simulink model "DR18E_Testpult"  (R2017a)
settings: Solver=ode1  StartTime=0.0  StopTime=Inf  FixedStep=0.001  RelTol=1e-3
PostLoadFcn:
  | , if any(exist('dsrtsu_mdlpostloadfcn', 'file') == [2, 3, 6]), try dsrtsu_mdlpostloadfcn('Execute', bdroot); catch fprintf('Error in PostLoadFcn (dsrtsu_mdlpostloadfcn) for model "%s":\n %s\n', bdroot, lasterr); end, end,
model workspace: external: MAT-File C:\Users\DeltaRacing\Documents\dSPACE\MABX_DR18E\Model\DR18E_MABX_Parameter.mat (data not in the file)
values from neighbouring files (symbols this model uses):
  am = 1/Ts    (= 1)    [DR18E_MABX_Parameter.m]
  bm = K/Ts    (= 0.05)    [DR18E_MABX_Parameter.m]
  cf = 41350    [DR18E_MABX_Parameter.m]
  cr = 41350    [DR18E_MABX_Parameter.m]
  Derating_HV_Battery_Kapa = 1    [DR18E_MABX_Parameter.m]
  Derating_Start_km = 16    [DR18E_MABX_Parameter.m]
  Drive_Mode = 0    [DR18E_MABX_Parameter.m]
  g = 1    [DR18E_MABX_Parameter.m]
  Gas_Modus = 2    [DR18E_MABX_Parameter.m]
  HV_Power_max = 80    [DR18E_MABX_Parameter.m]
  i_Getriebe = 3.3    [DR18E_MABX_Parameter.m]
  i_Lenkgetriebe = 4.32    [DR18E_MABX_Parameter.m]
  K_SET = 1    [DR18E_MABX_Parameter.m]
  Kapazitaet_HV_Battery_kWh = 6.6    [DR18E_MABX_Parameter.m]
  KW_T_Soll = 37    [DR18E_MABX_Parameter.m]
  lf = 1.2    [DR18E_MABX_Parameter.m]
  lr = 1.15    [DR18E_MABX_Parameter.m]
  m = mdriver + mvehicle    (= 310)    [DR18E_MABX_Parameter.m]
  M_max = 150    [DR18E_MABX_Parameter.m]
  Power_Limit_onoff = 0    [DR18E_MABX_Parameter.m]
  Reifenradius = 0.2351    [DR18E_MABX_Parameter.m]
  Strecke_Endu_km = 22    [DR18E_MABX_Parameter.m]
  TC_Decr_Gas = 0.00005    (= 5e-05)    [DR18E_MABX_Parameter.m]
  TC_Derivative = 0.4    [DR18E_MABX_Parameter.m]
  TC_Incr_Gas = 0.005    [DR18E_MABX_Parameter.m]
  TC_On = 0    [DR18E_MABX_Parameter.m]
  TC_Relay_Off = 0.065    [DR18E_MABX_Parameter.m]
  TC_Relay_On = 0.07    [DR18E_MABX_Parameter.m]
  TV_Mode = 2    [DR18E_MABX_Parameter.m]
  TV_On = 0    [DR18E_MABX_Parameter.m]
  TV_Override = 1    [DR18E_MABX_Parameter.m]
  y = 0.8    [DR18E_MABX_Parameter.m]
undefined symbols (not defined in the file or in its folder): D, DiscIntNeverNeededParam, I, K_OL, P
libraries: simulink x288, rtican x100, rtiusbflightreclib x40, rti1401lib_dio_type3 x10, simulink_extras x10, rti1401lib_adc_type4 x8, rti1401lib_II_base x7
(part 17 of 27)

== system DR18E_Testpult/Verarbeitung/Precalculations/FlightRecorder ==
  In1 : Inport
  Data Type Conversion : DataTypeConversion
  Gain : Gain
  USB_FLIGHT_REC_BL1 : rtiusbflightreclib/USB_FLIGHT_REC_BL1  VarName=v_kmh  DataType=Single  SampleTime=-1  TLCFileName=rtiusbflightrecwrite  Reserved1=[]  Reserved2=[]  Reserved3=[]  Reserved4=[]  DSProperties=struct('RTI',struct('Version',uint32(3),'BlockType',struct('isSLSource',uint8(0),'isSLSink',uint8(1),'isHWSource',uint8(0),'isHWSink',uint8(0),'isSetup',uint8(0),'isInline',uint8(1),'isNonInline',uint8(0),'isInterrupt',uint8(0),'isChannelwise',uint8(0)),'IOBoardType',{{'DSUSB','FLIGHTREC'}},'UnitType','FLIGHTREC','Identifier','WRITE','DialogType','SL','BlockSet','RTIUSBFLIGHTREC','SlaveProcessor','NONE'))  RTIBlockInterface=struct('InputPortsActive',1,'InputPortsWidth',int32(1),'InputPortsDataType',{{'SS_SINGLE'}},'BlockDisplay',{{['Write to\nUSB Flight Recorder'],'center'}},'IconTransparency','off','InitLevel',3,'BlockName',struct('Token',{{'USB_FLIGHT_REC_BL1'}}),'MaskDescription',['Write input to the Flight Recorder. Recorded data can be referenced by the specified variable.'],'SampleTime',{{-1}})  RTIBlockParameters=struct('VarName',{{'v_kmh','OFF',[]}},'DataType',{{'Single','OFF',[]}},'SampleTime',{{-1,'OFF',[]}},'TLCFileName',{{'rtiusbflightrecwrite','OFF',[]}})  RTISFcnParameters=struct('VarName','char','DataType','char','SampleTime','double','TLCFileName','char')  RTIBlockParaDefault=struct('VarName','Var1','DataType','Single','SampleTime',-1,'TLCFileName','rtiusbflightrecwrite')
      settings: SourceProductName=dSPACE RTI USB Flight Rec Blockset
  wires:
  Data Type Conversion/1 -> USB_FLIGHT_REC_BL1/1
  In1/1 -> Gain/1
  Gain/1 -> Data Type Conversion/1

== system DR18E_Testpult/Verarbeitung/Precalculations/FlightRecorder1 ==
  In1 : Inport
  Data Type Conversion : DataTypeConversion
  Gain : Gain
  USB_FLIGHT_REC_BL1 : rtiusbflightreclib/USB_FLIGHT_REC_BL1  VarName=DrehzahlRL_rpm  DataType=Single  SampleTime=-1  TLCFileName=rtiusbflightrecwrite  Reserved1=[]  Reserved2=[]  Reserved3=[]  Reserved4=[]  DSProperties=struct('RTI',struct('Version',uint32(3),'BlockType',struct('isSLSource',uint8(0),'isSLSink',uint8(1),'isHWSource',uint8(0),'isHWSink',uint8(0),'isSetup',uint8(0),'isInline',uint8(1),'isNonInline',uint8(0),'isInterrupt',uint8(0),'isChannelwise',uint8(0)),'IOBoardType',{{'DSUSB','FLIGHTREC'}},'UnitType','FLIGHTREC','Identifier','WRITE','DialogType','SL','BlockSet','RTIUSBFLIGHTREC','SlaveProcessor','NONE'))  RTIBlockInterface=struct('InputPortsActive',1,'InputPortsWidth',int32(1),'InputPortsDataType',{{'SS_SINGLE'}},'BlockDisplay',{{['Write to\nUSB Flight Recorder'],'center'}},'IconTransparency','off','InitLevel',3,'BlockName',struct('Token',{{'USB_FLIGHT_REC_BL1'}}),'MaskDescription',['Write input to the Flight Recorder. Recorded data can be referenced by the specified variable.'],'SampleTime',{{-1}})  RTIBlockParameters=struct('VarName',{{'DrehzahlRL_rpm','OFF',[]}},'DataType',{{'Single','OFF',[]}},'SampleTime',{{-1,'OFF',[]}},'TLCFileName',{{'rtiusbflightrecwrite','OFF',[]}})  RTISFcnParameters=struct('VarName','char','DataType','char','SampleTime','double','TLCFileName','char')  RTIBlockParaDefault=struct('VarName','Var1','DataType','Single','SampleTime',-1,'TLCFileName','rtiusbflightrecwrite')
      settings: SourceProductName=dSPACE RTI USB Flight Rec Blockset
  wires:
  Data Type Conversion/1 -> USB_FLIGHT_REC_BL1/1
  In1/1 -> Gain/1
  Gain/1 -> Data Type Conversion/1

== system DR18E_Testpult/Verarbeitung/Precalculations/FlightRecorder2 ==
  In1 : Inport
  Data Type Conversion : DataTypeConversion
  Gain : Gain
  USB_FLIGHT_REC_BL1 : rtiusbflightreclib/USB_FLIGHT_REC_BL1  VarName=DrehzahlRR_rpm  DataType=Single  SampleTime=-1  TLCFileName=rtiusbflightrecwrite  Reserved1=[]  Reserved2=[]  Reserved3=[]  Reserved4=[]  DSProperties=struct('RTI',struct('Version',uint32(3),'BlockType',struct('isSLSource',uint8(0),'isSLSink',uint8(1),'isHWSource',uint8(0),'isHWSink',uint8(0),'isSetup',uint8(0),'isInline',uint8(1),'isNonInline',uint8(0),'isInterrupt',uint8(0),'isChannelwise',uint8(0)),'IOBoardType',{{'DSUSB','FLIGHTREC'}},'UnitType','FLIGHTREC','Identifier','WRITE','DialogType','SL','BlockSet','RTIUSBFLIGHTREC','SlaveProcessor','NONE'))  RTIBlockInterface=struct('InputPortsActive',1,'InputPortsWidth',int32(1),'InputPortsDataType',{{'SS_SINGLE'}},'BlockDisplay',{{['Write to\nUSB Flight Recorder'],'center'}},'IconTransparency','off','InitLevel',3,'BlockName',struct('Token',{{'USB_FLIGHT_REC_BL1'}}),'MaskDescription',['Write input to the Flight Recorder. Recorded data can be referenced by the specified variable.'],'SampleTime',{{-1}})  RTIBlockParameters=struct('VarName',{{'DrehzahlRR_rpm','OFF',[]}},'DataType',{{'Single','OFF',[]}},'SampleTime',{{-1,'OFF',[]}},'TLCFileName',{{'rtiusbflightrecwrite','OFF',[]}})  RTISFcnParameters=struct('VarName','char','DataType','char','SampleTime','double','TLCFileName','char')  RTIBlockParaDefault=struct('VarName','Var1','DataType','Single','SampleTime',-1,'TLCFileName','rtiusbflightrecwrite')
      settings: SourceProductName=dSPACE RTI USB Flight Rec Blockset
  wires:
  Data Type Conversion/1 -> USB_FLIGHT_REC_BL1/1
  In1/1 -> Gain/1
  Gain/1 -> Data Type Conversion/1

== system DR18E_Testpult/Verarbeitung/Precalculations/FlightRecorder3 ==
  In1 : Inport
  Data Type Conversion : DataTypeConversion
  Gain : Gain
  USB_FLIGHT_REC_BL1 : rtiusbflightreclib/USB_FLIGHT_REC_BL1  VarName=DrehzahlFR_rpm  DataType=Single  SampleTime=-1  TLCFileName=rtiusbflightrecwrite  Reserved1=[]  Reserved2=[]  Reserved3=[]  Reserved4=[]  DSProperties=struct('RTI',struct('Version',uint32(3),'BlockType',struct('isSLSource',uint8(0),'isSLSink',uint8(1),'isHWSource',uint8(0),'isHWSink',uint8(0),'isSetup',uint8(0),'isInline',uint8(1),'isNonInline',uint8(0),'isInterrupt',uint8(0),'isChannelwise',uint8(0)),'IOBoardType',{{'DSUSB','FLIGHTREC'}},'UnitType','FLIGHTREC','Identifier','WRITE','DialogType','SL','BlockSet','RTIUSBFLIGHTREC','SlaveProcessor','NONE'))  RTIBlockInterface=struct('InputPortsActive',1,'InputPortsWidth',int32(1),'InputPortsDataType',{{'SS_SINGLE'}},'BlockDisplay',{{['Write to\nUSB Flight Recorder'],'center'}},'IconTransparency','off','InitLevel',3,'BlockName',struct('Token',{{'USB_FLIGHT_REC_BL1'}}),'MaskDescription',['Write input to the Flight Recorder. Recorded data can be referenced by the specified variable.'],'SampleTime',{{-1}})  RTIBlockParameters=struct('VarName',{{'DrehzahlFR_rpm','OFF',[]}},'DataType',{{'Single','OFF',[]}},'SampleTime',{{-1,'OFF',[]}},'TLCFileName',{{'rtiusbflightrecwrite','OFF',[]}})  RTISFcnParameters=struct('VarName','char','DataType','char','SampleTime','double','TLCFileName','char')  RTIBlockParaDefault=struct('VarName','Var1','DataType','Single','SampleTime',-1,'TLCFileName','rtiusbflightrecwrite')
      settings: SourceProductName=dSPACE RTI USB Flight Rec Blockset
  wires:
  Data Type Conversion/1 -> USB_FLIGHT_REC_BL1/1
  In1/1 -> Gain/1
  Gain/1 -> Data Type Conversion/1

== system DR18E_Testpult/Verarbeitung/Precalculations/FlightRecorder4 ==
  In1 : Inport
  Data Type Conversion : DataTypeConversion
  Gain : Gain
  USB_FLIGHT_REC_BL1 : rtiusbflightreclib/USB_FLIGHT_REC_BL1  VarName=DrehzahlFL_rpm  DataType=Single  SampleTime=-1  TLCFileName=rtiusbflightrecwrite  Reserved1=[]  Reserved2=[]  Reserved3=[]  Reserved4=[]  DSProperties=struct('RTI',struct('Version',uint32(3),'BlockType',struct('isSLSource',uint8(0),'isSLSink',uint8(1),'isHWSource',uint8(0),'isHWSink',uint8(0),'isSetup',uint8(0),'isInline',uint8(1),'isNonInline',uint8(0),'isInterrupt',uint8(0),'isChannelwise',uint8(0)),'IOBoardType',{{'DSUSB','FLIGHTREC'}},'UnitType','FLIGHTREC','Identifier','WRITE','DialogType','SL','BlockSet','RTIUSBFLIGHTREC','SlaveProcessor','NONE'))  RTIBlockInterface=struct('InputPortsActive',1,'InputPortsWidth',int32(1),'InputPortsDataType',{{'SS_SINGLE'}},'BlockDisplay',{{['Write to\nUSB Flight Recorder'],'center'}},'IconTransparency','off','InitLevel',3,'BlockName',struct('Token',{{'USB_FLIGHT_REC_BL1'}}),'MaskDescription',['Write input to the Flight Recorder. Recorded data can be referenced by the specified variable.'],'SampleTime',{{-1}})  RTIBlockParameters=struct('VarName',{{'DrehzahlFL_rpm','OFF',[]}},'DataType',{{'Single','OFF',[]}},'SampleTime',{{-1,'OFF',[]}},'TLCFileName',{{'rtiusbflightrecwrite','OFF',[]}})  RTISFcnParameters=struct('VarName','char','DataType','char','SampleTime','double','TLCFileName','char')  RTIBlockParaDefault=struct('VarName','Var1','DataType','Single','SampleTime',-1,'TLCFileName','rtiusbflightrecwrite')
      settings: SourceProductName=dSPACE RTI USB Flight Rec Blockset
  wires:
  Data Type Conversion/1 -> USB_FLIGHT_REC_BL1/1
  In1/1 -> Gain/1
  Gain/1 -> Data Type Conversion/1

== system DR18E_Testpult/Verarbeitung/Precalculations/FlightRecorder5 ==
  In1 : Inport
  Data Type Conversion : DataTypeConversion
  Gain : Gain
  USB_FLIGHT_REC_BL1 : rtiusbflightreclib/USB_FLIGHT_REC_BL1  VarName=slip_links_0_1  DataType=Single  SampleTime=-1  TLCFileName=rtiusbflightrecwrite  Reserved1=[]  Reserved2=[]  Reserved3=[]  Reserved4=[]  DSProperties=struct('RTI',struct('Version',uint32(3),'BlockType',struct('isSLSource',uint8(0),'isSLSink',uint8(1),'isHWSource',uint8(0),'isHWSink',uint8(0),'isSetup',uint8(0),'isInline',uint8(1),'isNonInline',uint8(0),'isInterrupt',uint8(0),'isChannelwise',uint8(0)),'IOBoardType',{{'DSUSB','FLIGHTREC'}},'UnitType','FLIGHTREC','Identifier','WRITE','DialogType','SL','BlockSet','RTIUSBFLIGHTREC','SlaveProcessor','NONE'))  RTIBlockInterface=struct('InputPortsActive',1,'InputPortsWidth',int32(1),'InputPortsDataType',{{'SS_SINGLE'}},'BlockDisplay',{{['Write to\nUSB Flight Recorder'],'center'}},'IconTransparency','off','InitLevel',3,'BlockName',struct('Token',{{'USB_FLIGHT_REC_BL1'}}),'MaskDescription',['Write input to the Flight Recorder. Recorded data can be referenced by the specified variable.'],'SampleTime',{{-1}})  RTIBlockParameters=struct('VarName',{{'slip_links_0_1','OFF',[]}},'DataType',{{'Single','OFF',[]}},'SampleTime',{{-1,'OFF',[]}},'TLCFileName',{{'rtiusbflightrecwrite','OFF',[]}})  RTISFcnParameters=struct('VarName','char','DataType','char','SampleTime','double','TLCFileName','char')  RTIBlockParaDefault=struct('VarName','Var1','DataType','Single','SampleTime',-1,'TLCFileName','rtiusbflightrecwrite')
      settings: SourceProductName=dSPACE RTI USB Flight Rec Blockset
  wires:
  Data Type Conversion/1 -> USB_FLIGHT_REC_BL1/1
  In1/1 -> Gain/1
  Gain/1 -> Data Type Conversion/1

== system DR18E_Testpult/Verarbeitung/Precalculations/FlightRecorder6 ==
  In1 : Inport
  Data Type Conversion : DataTypeConversion
  Gain : Gain
  USB_FLIGHT_REC_BL1 : rtiusbflightreclib/USB_FLIGHT_REC_BL1  VarName=slip_rechts_0_1  DataType=Single  SampleTime=-1  TLCFileName=rtiusbflightrecwrite  Reserved1=[]  Reserved2=[]  Reserved3=[]  Reserved4=[]  DSProperties=struct('RTI',struct('Version',uint32(3),'BlockType',struct('isSLSource',uint8(0),'isSLSink',uint8(1),'isHWSource',uint8(0),'isHWSink',uint8(0),'isSetup',uint8(0),'isInline',uint8(1),'isNonInline',uint8(0),'isInterrupt',uint8(0),'isChannelwise',uint8(0)),'IOBoardType',{{'DSUSB','FLIGHTREC'}},'UnitType','FLIGHTREC','Identifier','WRITE','DialogType','SL','BlockSet','RTIUSBFLIGHTREC','SlaveProcessor','NONE'))  RTIBlockInterface=struct('InputPortsActive',1,'InputPortsWidth',int32(1),'InputPortsDataType',{{'SS_SINGLE'}},'BlockDisplay',{{['Write to\nUSB Flight Recorder'],'center'}},'IconTransparency','off','InitLevel',3,'BlockName',struct('Token',{{'USB_FLIGHT_REC_BL1'}}),'MaskDescription',['Write input to the Flight Recorder. Recorded data can be referenced by the specified variable.'],'SampleTime',{{-1}})  RTIBlockParameters=struct('VarName',{{'slip_rechts_0_1','OFF',[]}},'DataType',{{'Single','OFF',[]}},'SampleTime',{{-1,'OFF',[]}},'TLCFileName',{{'rtiusbflightrecwrite','OFF',[]}})  RTISFcnParameters=struct('VarName','char','DataType','char','SampleTime','double','TLCFileName','char')  RTIBlockParaDefault=struct('VarName','Var1','DataType','Single','SampleTime',-1,'TLCFileName','rtiusbflightrecwrite')
      settings: SourceProductName=dSPACE RTI USB Flight Rec Blockset
  wires:
  Data Type Conversion/1 -> USB_FLIGHT_REC_BL1/1
  In1/1 -> Gain/1
  Gain/1 -> Data Type Conversion/1

== system DR18E_Testpult/Verarbeitung/Precalculations/kilometer tracking ==
  v_ms : Inport
  Discrete-Time Integrator : DiscreteIntegrator  SampleTime=-1  ICPrevOutput=DiscIntNeverNeededParam  ICPrevScaledInput=DiscIntNeverNeededParam
  FlightRecorder1 : Subsystem
  s_m : Gain
  tag scope: Tagesmeter_s_m=global
  wires:
  v_ms/1 -> Discrete-Time Integrator/1
  s_m/1 -> [Tagesmeter_s_m], FlightRecorder1/1(In1)  "Tagesmeter_fluechtig_s_m"
  Discrete-Time Integrator/1 -> s_m/1

== system DR18E_Testpult/Verarbeitung/Strom//SOC/HVIRecorder ==
  In1 : Inport
  Data Type Conversion : DataTypeConversion
  Gain : Gain
  USB_FLIGHT_REC_BL1 : rtiusbflightreclib/USB_FLIGHT_REC_BL1  VarName=HV_current_A  DataType=Single  SampleTime=-1  TLCFileName=rtiusbflightrecwrite  Reserved1=[]  Reserved2=[]  Reserved3=[]  Reserved4=[]  DSProperties=struct('RTI',struct('Version',uint32(3),'BlockType',struct('isSLSource',uint8(0),'isSLSink',uint8(1),'isHWSource',uint8(0),'isHWSink',uint8(0),'isSetup',uint8(0),'isInline',uint8(1),'isNonInline',uint8(0),'isInterrupt',uint8(0),'isChannelwise',uint8(0)),'IOBoardType',{{'DSUSB','FLIGHTREC'}},'UnitType','FLIGHTREC','Identifier','WRITE','DialogType','SL','BlockSet','RTIUSBFLIGHTREC','SlaveProcessor','NONE'))  RTIBlockInterface=struct('InputPortsActive',1,'InputPortsWidth',int32(1),'InputPortsDataType',{{'SS_SINGLE'}},'BlockDisplay',{{['Write to\nUSB Flight Recorder'],'center'}},'IconTransparency','off','InitLevel',3,'BlockName',struct('Token',{{'USB_FLIGHT_REC_BL1'}}),'MaskDescription',['Write input to the Flight Recorder. Recorded data can be referenced by the specified variable.'],'SampleTime',{{-1}})  RTIBlockParameters=struct('VarName',{{'HV_current_A','OFF',[]}},'DataType',{{'Single','OFF',[]}},'SampleTime',{{-1,'OFF',[]}},'TLCFileName',{{'rtiusbflightrecwrite','OFF',[]}})  RTISFcnParameters=struct('VarName','char','DataType','char','SampleTime','double','TLCFileName','char')  RTIBlockParaDefault=struct('VarName','Var1','DataType','Single','SampleTime',-1,'TLCFileName','rtiusbflightrecwrite')
      settings: SourceProductName=dSPACE RTI USB Flight Rec Blockset
  wires:
  Data Type Conversion/1 -> USB_FLIGHT_REC_BL1/1
  In1/1 -> Gain/1
  Gain/1 -> Data Type Conversion/1

== system DR18E_Testpult/Verarbeitung/Strom//SOC/HVURecorder ==
  In1 : Inport
  Data Type Conversion : DataTypeConversion
  Gain : Gain
  USB_FLIGHT_REC_BL1 : rtiusbflightreclib/USB_FLIGHT_REC_BL1  VarName=HV_voltage_V  DataType=Single  SampleTime=-1  TLCFileName=rtiusbflightrecwrite  Reserved1=[]  Reserved2=[]  Reserved3=[]  Reserved4=[]  DSProperties=struct('RTI',struct('Version',uint32(3),'BlockType',struct('isSLSource',uint8(0),'isSLSink',uint8(1),'isHWSource',uint8(0),'isHWSink',uint8(0),'isSetup',uint8(0),'isInline',uint8(1),'isNonInline',uint8(0),'isInterrupt',uint8(0),'isChannelwise',uint8(0)),'IOBoardType',{{'DSUSB','FLIGHTREC'}},'UnitType','FLIGHTREC','Identifier','WRITE','DialogType','SL','BlockSet','RTIUSBFLIGHTREC','SlaveProcessor','NONE'))  RTIBlockInterface=struct('InputPortsActive',1,'InputPortsWidth',int32(1),'InputPortsDataType',{{'SS_SINGLE'}},'BlockDisplay',{{['Write to\nUSB Flight Recorder'],'center'}},'IconTransparency','off','InitLevel',3,'BlockName',struct('Token',{{'USB_FLIGHT_REC_BL1'}}),'MaskDescription',['Write input to the Flight Recorder. Recorded data can be referenced by the specified variable.'],'SampleTime',{{-1}})  RTIBlockParameters=struct('VarName',{{'HV_voltage_V','OFF',[]}},'DataType',{{'Single','OFF',[]}},'SampleTime',{{-1,'OFF',[]}},'TLCFileName',{{'rtiusbflightrecwrite','OFF',[]}})  RTISFcnParameters=struct('VarName','char','DataType','char','SampleTime','double','TLCFileName','char')  RTIBlockParaDefault=struct('VarName','Var1','DataType','Single','SampleTime',-1,'TLCFileName','rtiusbflightrecwrite')
      settings: SourceProductName=dSPACE RTI USB Flight Rec Blockset
  wires:
  Data Type Conversion/1 -> USB_FLIGHT_REC_BL1/1
  In1/1 -> Gain/1
  Gain/1 -> Data Type Conversion/1

== system DR18E_Testpult/Verarbeitung/Strom//SOC/currentConsumptionRecorder ==
  In1 : Inport
  Data Type Conversion : DataTypeConversion
  Gain : Gain
  USB_FLIGHT_REC_BL1 : rtiusbflightreclib/USB_FLIGHT_REC_BL1  VarName=currentConsumption_As  DataType=Single  SampleTime=-1  TLCFileName=rtiusbflightrecwrite  Reserved1=[]  Reserved2=[]  Reserved3=[]  Reserved4=[]  DSProperties=struct('RTI',struct('Version',uint32(3),'BlockType',struct('isSLSource',uint8(0),'isSLSink',uint8(1),'isHWSource',uint8(0),'isHWSink',uint8(0),'isSetup',uint8(0),'isInline',uint8(1),'isNonInline',uint8(0),'isInterrupt',uint8(0),'isChannelwise',uint8(0)),'IOBoardType',{{'DSUSB','FLIGHTREC'}},'UnitType','FLIGHTREC','Identifier','WRITE','DialogType','SL','BlockSet','RTIUSBFLIGHTREC','SlaveProcessor','NONE'))  RTIBlockInterface=struct('InputPortsActive',1,'InputPortsWidth',int32(1),'InputPortsDataType',{{'SS_SINGLE'}},'BlockDisplay',{{['Write to\nUSB Flight Recorder'],'center'}},'IconTransparency','off','InitLevel',3,'BlockName',struct('Token',{{'USB_FLIGHT_REC_BL1'}}),'MaskDescription',['Write input to the Flight Recorder. Recorded data can be referenced by the specified variable.'],'SampleTime',{{-1}})  RTIBlockParameters=struct('VarName',{{'currentConsumption_As','OFF',[]}},'DataType',{{'Single','OFF',[]}},'SampleTime',{{-1,'OFF',[]}},'TLCFileName',{{'rtiusbflightrecwrite','OFF',[]}})  RTISFcnParameters=struct('VarName','char','DataType','char','SampleTime','double','TLCFileName','char')  RTIBlockParaDefault=struct('VarName','Var1','DataType','Single','SampleTime',-1,'TLCFileName','rtiusbflightrecwrite')
      settings: SourceProductName=dSPACE RTI USB Flight Rec Blockset
  wires:
  Data Type Conversion/1 -> USB_FLIGHT_REC_BL1/1
  In1/1 -> Gain/1
  Gain/1 -> Data Type Conversion/1

== system DR18E_Testpult/Verarbeitung/Strom//SOC/powerConsumtionRecorder ==
  In1 : Inport
  Data Type Conversion : DataTypeConversion
  Gain : Gain
  USB_FLIGHT_REC_BL1 : rtiusbflightreclib/USB_FLIGHT_REC_BL1  VarName=powerConsumption_Ws  DataType=Single  SampleTime=-1  TLCFileName=rtiusbflightrecwrite  Reserved1=[]  Reserved2=[]  Reserved3=[]  Reserved4=[]  DSProperties=struct('RTI',struct('Version',uint32(3),'BlockType',struct('isSLSource',uint8(0),'isSLSink',uint8(1),'isHWSource',uint8(0),'isHWSink',uint8(0),'isSetup',uint8(0),'isInline',uint8(1),'isNonInline',uint8(0),'isInterrupt',uint8(0),'isChannelwise',uint8(0)),'IOBoardType',{{'DSUSB','FLIGHTREC'}},'UnitType','FLIGHTREC','Identifier','WRITE','DialogType','SL','BlockSet','RTIUSBFLIGHTREC','SlaveProcessor','NONE'))  RTIBlockInterface=struct('InputPortsActive',1,'InputPortsWidth',int32(1),'InputPortsDataType',{{'SS_SINGLE'}},'BlockDisplay',{{['Write to\nUSB Flight Recorder'],'center'}},'IconTransparency','off','InitLevel',3,'BlockName',struct('Token',{{'USB_FLIGHT_REC_BL1'}}),'MaskDescription',['Write input to the Flight Recorder. Recorded data can be referenced by the specified variable.'],'SampleTime',{{-1}})  RTIBlockParameters=struct('VarName',{{'powerConsumption_Ws','OFF',[]}},'DataType',{{'Single','OFF',[]}},'SampleTime',{{-1,'OFF',[]}},'TLCFileName',{{'rtiusbflightrecwrite','OFF',[]}})  RTISFcnParameters=struct('VarName','char','DataType','char','SampleTime','double','TLCFileName','char')  RTIBlockParaDefault=struct('VarName','Var1','DataType','Single','SampleTime',-1,'TLCFileName','rtiusbflightrecwrite')
      settings: SourceProductName=dSPACE RTI USB Flight Rec Blockset
  wires:
  Data Type Conversion/1 -> USB_FLIGHT_REC_BL1/1
  In1/1 -> Gain/1
  Gain/1 -> Data Type Conversion/1

== system DR18E_Testpult/Verarbeitung/Strom//SOC/powerRecorder ==
  In1 : Inport
  Data Type Conversion : DataTypeConversion
  Gain : Gain
  USB_FLIGHT_REC_BL1 : rtiusbflightreclib/USB_FLIGHT_REC_BL1  VarName=HV_power_W  DataType=Single  SampleTime=-1  TLCFileName=rtiusbflightrecwrite  Reserved1=[]  Reserved2=[]  Reserved3=[]  Reserved4=[]  DSProperties=struct('RTI',struct('Version',uint32(3),'BlockType',struct('isSLSource',uint8(0),'isSLSink',uint8(1),'isHWSource',uint8(0),'isHWSink',uint8(0),'isSetup',uint8(0),'isInline',uint8(1),'isNonInline',uint8(0),'isInterrupt',uint8(0),'isChannelwise',uint8(0)),'IOBoardType',{{'DSUSB','FLIGHTREC'}},'UnitType','FLIGHTREC','Identifier','WRITE','DialogType','SL','BlockSet','RTIUSBFLIGHTREC','SlaveProcessor','NONE'))  RTIBlockInterface=struct('InputPortsActive',1,'InputPortsWidth',int32(1),'InputPortsDataType',{{'SS_SINGLE'}},'BlockDisplay',{{['Write to\nUSB Flight Recorder'],'center'}},'IconTransparency','off','InitLevel',3,'BlockName',struct('Token',{{'USB_FLIGHT_REC_BL1'}}),'MaskDescription',['Write input to the Flight Recorder. Recorded data can be referenced by the specified variable.'],'SampleTime',{{-1}})  RTIBlockParameters=struct('VarName',{{'HV_power_W','OFF',[]}},'DataType',{{'Single','OFF',[]}},'SampleTime',{{-1,'OFF',[]}},'TLCFileName',{{'rtiusbflightrecwrite','OFF',[]}})  RTISFcnParameters=struct('VarName','char','DataType','char','SampleTime','double','TLCFileName','char')  RTIBlockParaDefault=struct('VarName','Var1','DataType','Single','SampleTime',-1,'TLCFileName','rtiusbflightrecwrite')
      settings: SourceProductName=dSPACE RTI USB Flight Rec Blockset
  wires:
  Data Type Conversion/1 -> USB_FLIGHT_REC_BL1/1
  In1/1 -> Gain/1
  Gain/1 -> Data Type Conversion/1

== system DR18E_Testpult/Verarbeitung/Temperaturregelung1/Detect Max Temp ==
  STK 1-5 : Inport
  STK 6-10 : Inport  Port=2
  Bus Selector : BusSelector  OutputSignals=STK1_Temp1-5.STK1_Temp1,STK1_Temp1-5.STK1_Temp2,STK1_Temp1-5.STK1_Temp3,STK1_Temp1-5.STK1_Temp4,STK1_Temp1-5.STK1_Temp5,STK2_Temp1-5.STK2_Temp1,STK2_Temp1-5.STK2_Temp2,STK2_Temp1-5.STK2_Temp3,STK2_Temp1-5.STK2_Temp4,STK2_Temp1-5.STK2_Temp5,STK3_Temp1-5.STK3_Temp1,STK3_Temp1-5.STK3_Temp2,STK3_Temp1-5.STK3_Temp3,STK3_Temp1-5.STK3_Temp4,STK3_Temp1-5.STK3_Temp5,STK4_Temp1-5.STK4_Temp1,STK4_Temp1-5.STK4_Temp2,STK4_Temp1-5.STK4_Temp3,STK4_Temp1-5.STK4_Temp4,STK4_Temp1-5.STK4_Temp5,STK5_Temp1-5.STK5_Temp1,STK5_Temp1-5.STK5_Temp2,STK5_Temp1-5.STK5_Temp3,STK5_Temp1-5.STK5_Temp4,STK5_Temp1-5.STK5_Temp5
  Bus Selector1 : BusSelector  OutputSignals=STK6_Temp1-5.STK6_Temp1,STK6_Temp1-5.STK6_Temp2,STK6_Temp1-5.STK6_Temp3,STK6_Temp1-5.STK6_Temp4,STK6_Temp1-5.STK6_Temp5,STK7_Temp1-5.STK7_Temp1,STK7_Temp1-5.STK7_Temp2,STK7_Temp1-5.STK7_Temp3,STK7_Temp1-5.STK7_Temp4,STK7_Temp1-5.STK7_Temp5,STK8_Temp1-5.STK8_Temp1,STK8_Temp1-5.STK8_Temp2,STK8_Temp1-5.STK8_Temp3,STK8_Temp1-5.STK8_Temp4,STK8_Temp1-5.STK8_Temp5,STK9_Temp1-5.STK9_Temp1,STK9_Temp1-5.STK9_Temp2,STK9_Temp1-5.STK9_Temp3,STK9_Temp1-5.STK9_Temp4,STK9_Temp1-5.STK9_Temp5,STK10_Temp1-5.STK10_Temp1,STK10_Temp1-5.STK10_Temp2,STK10_Temp1-5.STK10_Temp3,STK10_Temp1-5.STK10_Temp4,STK10_Temp1-5.STK10_Temp5
  MinMax : MinMax  Function=max  Inputs=25
  MinMax1 : MinMax  Function=max  Inputs=25
  MinMax2 : MinMax  Function=max  Inputs=2
  HV Battery Max Temp : Outport
  wires:
  STK 1-5/1 -> Bus Selector/1
  Bus Selector/25 -> MinMax/25  "<STK5_Temp5>"
  Bus Selector/24 -> MinMax/24  "<STK5_Temp4>"
  Bus Selector/23 -> MinMax/23  "<STK5_Temp3>"
  Bus Selector/22 -> MinMax/22  "<STK5_Temp2>"
  Bus Selector/21 -> MinMax/21  "<STK5_Temp1>"
  Bus Selector/20 -> MinMax/20  "<STK4_Temp5>"
  Bus Selector/19 -> MinMax/19  "<STK4_Temp4>"
  Bus Selector/18 -> MinMax/18  "<STK4_Temp3>"
  Bus Selector/17 -> MinMax/17  "<STK4_Temp2>"
  Bus Selector/16 -> MinMax/16  "<STK4_Temp1>"
  Bus Selector/15 -> MinMax/15  "<STK3_Temp5>"
  Bus Selector/14 -> MinMax/14  "<STK3_Temp4>"
  Bus Selector/13 -> MinMax/13  "<STK3_Temp3>"
  Bus Selector/12 -> MinMax/12  "<STK3_Temp2>"
  Bus Selector/11 -> MinMax/11  "<STK3_Temp1>"
  Bus Selector/10 -> MinMax/10  "<STK2_Temp5>"
  Bus Selector/9 -> MinMax/9  "<STK2_Temp4>"
  Bus Selector/8 -> MinMax/8  "<STK2_Temp3>"
  Bus Selector/7 -> MinMax/7  "<STK2_Temp2>"
  Bus Selector/6 -> MinMax/6  "<STK2_Temp1>"
  Bus Selector/5 -> MinMax/5  "<STK1_Temp5>"
  Bus Selector/4 -> MinMax/4  "<STK1_Temp4>"
  Bus Selector/3 -> MinMax/3  "<STK1_Temp3>"
  Bus Selector/2 -> MinMax/2  "<STK1_Temp2>"
  Bus Selector/1 -> MinMax/1  "<STK1_Temp1>"
  MinMax2/1 -> HV Battery Max Temp/1
  MinMax/1 -> MinMax2/1
  Bus Selector1/20 -> MinMax1/20  "<STK9_Temp5>"
  Bus Selector1/21 -> MinMax1/21  "<STK10_Temp1>"
  Bus Selector1/23 -> MinMax1/23  "<STK10_Temp3>"
  Bus Selector1/19 -> MinMax1/19  "<STK9_Temp4>"
  Bus Selector1/22 -> MinMax1/22  "<STK10_Temp2>"
  Bus Selector1/24 -> MinMax1/24  "<STK10_Temp4>"
  MinMax1/1 -> MinMax2/2
  STK 6-10/1 -> Bus Selector1/1
  Bus Selector1/1 -> MinMax1/1  "<STK6_Temp1>"
  Bus Selector1/2 -> MinMax1/2  "<STK6_Temp2>"
  Bus Selector1/3 -> MinMax1/3  "<STK6_Temp3>"
  Bus Selector1/4 -> MinMax1/4  "<STK6_Temp4>"
  Bus Selector1/5 -> MinMax1/5  "<STK6_Temp5>"
  Bus Selector1/6 -> MinMax1/6  "<STK7_Temp1>"
  Bus Selector1/7 -> MinMax1/7  "<STK7_Temp2>"
  Bus Selector1/8 -> MinMax1/8  "<STK7_Temp3>"
  Bus Selector1/9 -> MinMax1/9  "<STK7_Temp4>"
  Bus Selector1/10 -> MinMax1/10  "<STK7_Temp5>"
  Bus Selector1/11 -> MinMax1/11  "<STK8_Temp1>"
  Bus Selector1/12 -> MinMax1/12  "<STK8_Temp2>"
  Bus Selector1/13 -> MinMax1/13  "<STK8_Temp3>"
  Bus Selector1/14 -> MinMax1/14  "<STK8_Temp4>"
  Bus Selector1/15 -> MinMax1/15  "<STK8_Temp5>"
  Bus Selector1/16 -> MinMax1/16  "<STK9_Temp1>"
  Bus Selector1/17 -> MinMax1/17  "<STK9_Temp2>"
  Bus Selector1/18 -> MinMax1/18  "<STK9_Temp3>"
  Bus Selector1/25 -> MinMax1/25  "<STK10_Temp5>"

== system DR18E_Testpult/Verarbeitung/Temperaturregelung1/ModeSelect ==
  Man/Aut Pulse : Inport
  Value Man : Inport  Port=2
  Value Aut : Inport  Port=3
  Constant : Constant  OutDataTypeStr=Inherit: Inherit via back propagation
  Data Type Conversion : DataTypeConversion  OutDataTypeStr=boolean
  J-K Flip-Flop : simulink_extras/Flip Flops/J-K Flip-Flop  initial_condition=0
      settings: SourceProductName=Simulink
  Switch : Switch  Criteria=u2 > Threshold
  Value : Outport
  wires:
  Value Man/1 -> Switch/1
  Value Aut/1 -> Switch/3
  Switch/1 -> Value/1
  Constant/1 -> J-K Flip-Flop/3, J-K Flip-Flop/1
  Man/Aut Pulse/1 -> Data Type Conversion/1
  J-K Flip-Flop/1 -> Switch/2  "Man/!Aut"
  Data Type Conversion/1 -> J-K Flip-Flop/2

== system DR18E_Testpult/Verarbeitung/Temperaturregelung1/ModeSelect1 ==
  Man/Aut Pulse : Inport
  Value Man : Inport  Port=2
  Value Aut : Inport  Port=3
  Constant : Constant  OutDataTypeStr=Inherit: Inherit via back propagation
  Data Type Conversion : DataTypeConversion  OutDataTypeStr=boolean
  J-K Flip-Flop : simulink_extras/Flip Flops/J-K Flip-Flop  initial_condition=0
      settings: SourceProductName=Simulink
  Switch : Switch  Criteria=u2 > Threshold
  Value : Outport
  wires:
  Value Man/1 -> Switch/1
  Value Aut/1 -> Switch/3
  Switch/1 -> Value/1
  Constant/1 -> J-K Flip-Flop/3, J-K Flip-Flop/1
  Man/Aut Pulse/1 -> Data Type Conversion/1
  J-K Flip-Flop/1 -> Switch/2  "Man/!Aut"
  Data Type Conversion/1 -> J-K Flip-Flop/2

== system DR18E_Testpult/Verarbeitung/Temperaturregelung1/ModeSelect2 ==
  Man/Aut Pulse : Inport
  Value Man : Inport  Port=2
  Value Aut : Inport  Port=3
  Constant : Constant  OutDataTypeStr=Inherit: Inherit via back propagation
  Data Type Conversion : DataTypeConversion  OutDataTypeStr=boolean
  J-K Flip-Flop : simulink_extras/Flip Flops/J-K Flip-Flop  initial_condition=0
      settings: SourceProductName=Simulink
  Switch : Switch  Criteria=u2 > Threshold
  Value : Outport
  wires:
  Value Man/1 -> Switch/1
  Value Aut/1 -> Switch/3
  Switch/1 -> Value/1
  Constant/1 -> J-K Flip-Flop/3, J-K Flip-Flop/1
  Man/Aut Pulse/1 -> Data Type Conversion/1
  J-K Flip-Flop/1 -> Switch/2  "Man/!Aut"
  Data Type Conversion/1 -> J-K Flip-Flop/2

== system DR18E_Testpult/Verarbeitung/Temperaturregelung1/PT1 Discrete ==
  u : Inport
  K : Inport  Port=2
  T : Inport  Port=3
  Memory : Memory
  Product : Product
  Product1 : Product
  Subsystem : Subsystem
  Sum : Sum  Inputs=|+-
  Sum1 : Sum  Inputs=|++
  y : Outport
  wires:
  K/1 -> Product/1
  Subsystem/1(T*) -> Product1/1
  u/1 -> Product/2
  Sum/1 -> Product1/2
  Product1/1 -> Sum1/1
  Memory/1 -> Sum1/2, Sum/2
  Sum1/1 -> y/1, Memory/1
  Product/1 -> Sum/1
  T/1 -> Subsystem/1(T)

== system DR18E_Testpult/Verarbeitung/Temperaturregelung1/PT1 Discrete1 ==
  u : Inport
  K : Inport  Port=2
  T : Inport  Port=3
  Memory : Memory
  Product : Product
  Product1 : Product
  Subsystem : Subsystem
  Sum : Sum  Inputs=|+-
  Sum1 : Sum  Inputs=|++
  y : Outport
  wires:
  K/1 -> Product/1
  Subsystem/1(T*) -> Product1/1
  u/1 -> Product/2
  Sum/1 -> Product1/2
  Product1/1 -> Sum1/1
  Memory/1 -> Sum1/2, Sum/2
  Sum1/1 -> y/1, Memory/1
  Product/1 -> Sum/1
  T/1 -> Subsystem/1(T)

== system DR18E_Testpult/Verarbeitung/Umrichter Init Config/Umrichter 1 Init Config ==
  note: TX-Register
  note: TX-Intervallzeit in ms
  Bus Creator : BusCreator  Inputs=8
  Bus Creator1 : BusCreator  Inputs=8
  TXReg1 : Constant  Value=hex2dec('30')  OutDataTypeStr=uint16
  TXReg2 : Constant  Value=hex2dec('27')  OutDataTypeStr=uint16
  TXReg3 : Constant  Value=hex2dec('49')  OutDataTypeStr=uint16
  TXReg4 : Constant  Value=hex2dec('90')  OutDataTypeStr=uint16
  TXReg5 : Constant  Value=hex2dec('40')  OutDataTypeStr=uint16
  TXReg6 : Constant  Value=hex2dec('8F')  OutDataTypeStr=uint16
  TXReg7 : Constant  Value=hex2dec('EB')  OutDataTypeStr=uint16
  TXReg8 : Constant  Value=hex2dec('4A')  OutDataTypeStr=uint16
  TXZeit1 : Constant  Value=127  OutDataTypeStr=uint16
  TXZeit2 : Constant  Value=129  OutDataTypeStr=uint16
  TXZeit3 : Constant  Value=254  OutDataTypeStr=uint16
  TXZeit4 : Constant  Value=113  OutDataTypeStr=uint16
  TXZeit5 : Constant  Value=105  OutDataTypeStr=uint16
  TXZeit6 : Constant  Value=131  OutDataTypeStr=uint16
  TXZeit7 : Constant  Value=254  OutDataTypeStr=uint16
  TXZeit8 : Constant  Value=254  OutDataTypeStr=uint16
  tag scope: U1config_TXRegister=global, U1config_TXZeiten=global
  wires:
  Bus Creator/1 -> [U1config_TXRegister]
  TXReg1/1 -> Bus Creator/1  "Drehzahl Istwert"
  TXReg2/1 -> Bus Creator/2  "Drehmoment Istwert"
  TXReg3/1 -> Bus Creator/3  "Motortemp"
  TXReg4/1 -> Bus Creator/4  "DrehmomentSollwert"
  TXReg5/1 -> Bus Creator/5  "Statusmeldung"
  TXReg6/1 -> Bus Creator/6  "Errormeldung"
  TXReg7/1 -> Bus Creator/7  "U_DC"
  TXReg8/1 -> Bus Creator/8  "InverterTemp"
  Bus Creator1/1 -> [U1config_TXZeiten]
  TXZeit1/1 -> Bus Creator1/1
  TXZeit2/1 -> Bus Creator1/2
  TXZeit3/1 -> Bus Creator1/3
  TXZeit4/1 -> Bus Creator1/4
  TXZeit5/1 -> Bus Creator1/5
  TXZeit6/1 -> Bus Creator1/6
  TXZeit7/1 -> Bus Creator1/7
  TXZeit8/1 -> Bus Creator1/8

== system DR18E_Testpult/Verarbeitung/Umrichter Init Config/Umrichter 2 Init Config ==
  note: TX-Register
  note: TX-Intervallzeit in ms
  Bus Creator : BusCreator  Inputs=8
  Bus Creator1 : BusCreator  Inputs=8
  TXReg1 : Constant  Value=hex2dec('30')  OutDataTypeStr=uint16
  TXReg2 : Constant  Value=hex2dec('27')  OutDataTypeStr=uint16
  TXReg3 : Constant  Value=hex2dec('49')  OutDataTypeStr=uint16
  TXReg4 : Constant  Value=hex2dec('90')  OutDataTypeStr=uint16
  TXReg5 : Constant  Value=hex2dec('40')  OutDataTypeStr=uint16
  TXReg6 : Constant  Value=hex2dec('8F')  OutDataTypeStr=uint16
  TXReg7 : Constant  Value=hex2dec('EB')  OutDataTypeStr=uint16
  TXReg8 : Constant  Value=hex2dec('4A')  OutDataTypeStr=uint16
  TXZeit1 : Constant  Value=127  OutDataTypeStr=uint16
  TXZeit2 : Constant  Value=134  OutDataTypeStr=uint16
  TXZeit3 : Constant  Value=254  OutDataTypeStr=uint16
  TXZeit4 : Constant  Value=109  OutDataTypeStr=uint16
  TXZeit5 : Constant  Value=131  OutDataTypeStr=uint16
  TXZeit6 : Constant  Value=103  OutDataTypeStr=uint16
  TXZeit7 : Constant  Value=254  OutDataTypeStr=uint16
  TXZeit8 : Constant  Value=254  OutDataTypeStr=uint16
  tag scope: U2config_TXRegister=global, U2config_TXZeiten=global
  wires:
  Bus Creator/1 -> [U2config_TXRegister]
  TXReg1/1 -> Bus Creator/1  "Drehzahl Istwert"
  TXReg2/1 -> Bus Creator/2  "Drehmoment Istwert"
  TXReg3/1 -> Bus Creator/3  "Motortemp"
  TXReg4/1 -> Bus Creator/4  "DrehmomentSollwert"
  TXReg5/1 -> Bus Creator/5  "Statusmeldung"
  TXReg6/1 -> Bus Creator/6  "Errormeldung"
  TXReg7/1 -> Bus Creator/7  "U_DC"
  TXReg8/1 -> Bus Creator/8  "InverterTemp"
  Bus Creator1/1 -> [U2config_TXZeiten]
  TXZeit1/1 -> Bus Creator1/1
  TXZeit2/1 -> Bus Creator1/2
  TXZeit3/1 -> Bus Creator1/3
  TXZeit4/1 -> Bus Creator1/4
  TXZeit5/1 -> Bus Creator1/5
  TXZeit6/1 -> Bus Creator1/6
  TXZeit7/1 -> Bus Creator1/7
  TXZeit8/1 -> Bus Creator1/8

== system DR18E_Testpult/Verarbeitung/Vehicle State Machine/FlightRecorder ==
  In1 : Inport
  Data Type Conversion : DataTypeConversion
  Gain : Gain
  USB_FLIGHT_REC_BL1 : rtiusbflightreclib/USB_FLIGHT_REC_BL1  VarName=State  DataType=Single  SampleTime=-1  TLCFileName=rtiusbflightrecwrite  Reserved1=[]  Reserved2=[]  Reserved3=[]  Reserved4=[]  DSProperties=struct('RTI',struct('Version',uint32(3),'BlockType',struct('isSLSource',uint8(0),'isSLSink',uint8(1),'isHWSource',uint8(0),'isHWSink',uint8(0),'isSetup',uint8(0),'isInline',uint8(1),'isNonInline',uint8(0),'isInterrupt',uint8(0),'isChannelwise',uint8(0)),'IOBoardType',{{'DSUSB','FLIGHTREC'}},'UnitType','FLIGHTREC','Identifier','WRITE','DialogType','SL','BlockSet','RTIUSBFLIGHTREC','SlaveProcessor','NONE'))  RTIBlockInterface=struct('InputPortsActive',1,'InputPortsWidth',int32(1),'InputPortsDataType',{{'SS_SINGLE'}},'BlockDisplay',{{['Write to\nUSB Flight Recorder'],'center'}},'IconTransparency','off','InitLevel',3,'BlockName',struct('Token',{{'USB_FLIGHT_REC_BL1'}}),'MaskDescription',['Write input to the Flight Recorder. Recorded data can be referenced by the specified variable.'],'SampleTime',{{-1}})  RTIBlockParameters=struct('VarName',{{'State','OFF',[]}},'DataType',{{'Single','OFF',[]}},'SampleTime',{{-1,'OFF',[]}},'TLCFileName',{{'rtiusbflightrecwrite','OFF',[]}})  RTISFcnParameters=struct('VarName','char','DataType','char','SampleTime','double','TLCFileName','char')  RTIBlockParaDefault=struct('VarName','Var1','DataType','Single','SampleTime',-1,'TLCFileName','rtiusbflightrecwrite')
      settings: SourceProductName=dSPACE RTI USB Flight Rec Blockset
  wires:
  Data Type Conversion/1 -> USB_FLIGHT_REC_BL1/1
  In1/1 -> Gain/1
  Gain/1 -> Data Type Conversion/1

== system DR18E_Testpult/Verarbeitung/Vehicle State Machine/FlightRecorder1 ==
  In1 : Inport
  Data Type Conversion : DataTypeConversion
  Gain : Gain
  USB_FLIGHT_REC_BL1 : rtiusbflightreclib/USB_FLIGHT_REC_BL1  VarName=ErrorNo  DataType=Single  SampleTime=-1  TLCFileName=rtiusbflightrecwrite  Reserved1=[]  Reserved2=[]  Reserved3=[]  Reserved4=[]  DSProperties=struct('RTI',struct('Version',uint32(3),'BlockType',struct('isSLSource',uint8(0),'isSLSink',uint8(1),'isHWSource',uint8(0),'isHWSink',uint8(0),'isSetup',uint8(0),'isInline',uint8(1),'isNonInline',uint8(0),'isInterrupt',uint8(0),'isChannelwise',uint8(0)),'IOBoardType',{{'DSUSB','FLIGHTREC'}},'UnitType','FLIGHTREC','Identifier','WRITE','DialogType','SL','BlockSet','RTIUSBFLIGHTREC','SlaveProcessor','NONE'))  RTIBlockInterface=struct('InputPortsActive',1,'InputPortsWidth',int32(1),'InputPortsDataType',{{'SS_SINGLE'}},'BlockDisplay',{{['Write to\nUSB Flight Recorder'],'center'}},'IconTransparency','off','InitLevel',3,'BlockName',struct('Token',{{'USB_FLIGHT_REC_BL1'}}),'MaskDescription',['Write input to the Flight Recorder. Recorded data can be referenced by the specified variable.'],'SampleTime',{{-1}})  RTIBlockParameters=struct('VarName',{{'ErrorNo','OFF',[]}},'DataType',{{'Single','OFF',[]}},'SampleTime',{{-1,'OFF',[]}},'TLCFileName',{{'rtiusbflightrecwrite','OFF',[]}})  RTISFcnParameters=struct('VarName','char','DataType','char','SampleTime','double','TLCFileName','char')  RTIBlockParaDefault=struct('VarName','Var1','DataType','Single','SampleTime',-1,'TLCFileName','rtiusbflightrecwrite')
      settings: SourceProductName=dSPACE RTI USB Flight Rec Blockset
  wires:
  Data Type Conversion/1 -> USB_FLIGHT_REC_BL1/1
  In1/1 -> Gain/1
  Gain/1 -> Data Type Conversion/1

== system DR18E_Testpult/Ausgabe/Inverter TX/Inverters TXTorque/TorqueMessage ==
  RegID_L_R : Inport
  Value32_L_R : Inport  Port=2
  Demux : Demux  Outputs=2
  Demux1 : Demux  Outputs=2
  U1_RegID : Outport
  U1_Value32 : Outport  Port=2
  U2_RegID : Outport  Port=3
  U2_Value32 : Outport  Port=4
  wires:
  Demux/2 -> U2_Value32/1
  Demux/1 -> U1_Value32/1
  Value32_L_R/1 -> Demux/1
  Demux1/1 -> U1_RegID/1
  Demux1/2 -> U2_RegID/1
  RegID_L_R/1 -> Demux1/1

== system DR18E_Testpult/Ausgabe/Inverter TX/Inverters TXUniversal/TorqueMessage ==
  RegID_L_R : Inport
  Value32_L_R : Inport  Port=2
  Demux : Demux  Outputs=2
  Demux1 : Demux  Outputs=2
  U1_RegID : Outport
  U1_Value32 : Outport  Port=2
  U2_RegID : Outport  Port=3
  U2_Value32 : Outport  Port=4
  wires:
  Demux/2 -> U2_Value32/1
  Demux/1 -> U1_Value32/1
  Value32_L_R/1 -> Demux/1
  Demux1/1 -> U1_RegID/1
  Demux1/2 -> U2_RegID/1
  RegID_L_R/1 -> Demux1/1

== system DR18E_Testpult/Ausgabe/Inverter TX/Inverters TXUniversal/Transmit OK Detection1 ==
  note: This subsystem surveys if the sending of the TX message is successful and if it meets the
      | requirements concerning the regularity of the sending.
      |
      | If for 5 consecutive execution steps the message could not be successfully sent the 'TX Warn'
      | output is set to 1. Also, the message is expected to be sent every 50 ms approximatively. If this
      | condition is not met 5 times consecutively the 'TX Warn' output is set to 1.
  TX status : Inport
  TX delta time : Inport  Port=2
  Delta time limit : Constant  Value=0.055
  Delta time limit exceeded : RelationalOperator  RndMeth=Nearest  InputSameDT=on
  Mem{1..4} (4 alike) : Memory
  OR : Logic  Operator=OR
  Prev. msg. not sent : RelationalOperator  Operator=~=  RndMeth=Nearest  InputSameDT=on
  Prev. msg. sent value : Constant
  Warn : Logic  Inputs=5
  TX Warn : Outport
  wires:
  TX delta time/1 -> Delta time limit exceeded/1
  Delta time limit/1 -> Delta time limit exceeded/2
  Prev. msg. sent value/1 -> Prev. msg. not sent/2
  TX status/1 -> Prev. msg. not sent/1
  Prev. msg. not sent/1 -> OR/1
  Delta time limit exceeded/1 -> OR/2
  OR/1 -> Mem1/1, Warn/1
  Mem1/1 -> Mem2/1, Warn/2
  Mem2/1 -> Mem3/1, Warn/3
  Mem3/1 -> Mem4/1, Warn/4
  Mem4/1 -> Warn/5
  Warn/1 -> TX Warn/1

== system DR18E_Testpult/Ausgabe/Inverter TX/Inverters TXUniversal/Transmit OK Detection2 ==
  note: This subsystem surveys if the sending of the TX message is successful and if it meets the
      | requirements concerning the regularity of the sending.
      |
      | If for 5 consecutive execution steps the message could not be successfully sent the 'TX Warn'
      | output is set to 1. Also, the message is expected to be sent every 50 ms approximatively. If this
      | condition is not met 5 times consecutively the 'TX Warn' output is set to 1.
  TX status : Inport
  TX delta time : Inport  Port=2
  Delta time limit : Constant  Value=0.055
  Delta time limit exceeded : RelationalOperator  RndMeth=Nearest  InputSameDT=on
  Mem{1..4} (4 alike) : Memory
  OR : Logic  Operator=OR
  Prev. msg. not sent : RelationalOperator  Operator=~=  RndMeth=Nearest  InputSameDT=on
  Prev. msg. sent value : Constant
  Warn : Logic  Inputs=5
  TX Warn : Outport
  wires:
  TX delta time/1 -> Delta time limit exceeded/1
  Delta time limit/1 -> Delta time limit exceeded/2
  Prev. msg. sent value/1 -> Prev. msg. not sent/2
  TX status/1 -> Prev. msg. not sent/1
  Prev. msg. not sent/1 -> OR/1
  Delta time limit exceeded/1 -> OR/2
  OR/1 -> Mem1/1, Warn/1
  Mem1/1 -> Mem2/1, Warn/2
  Mem2/1 -> Mem3/1, Warn/3
  Mem3/1 -> Mem4/1, Warn/4
  Mem4/1 -> Warn/5
  Warn/1 -> TX Warn/1

== system DR18E_Testpult/Ausgabe/Inverter TX/Umrichter Init/Transmit OK Detection ==
  note: This subsystem surveys if the sending of the TX message is successful and if it meets the
      | requirements concerning the regularity of the sending.
      |
      | If for 5 consecutive execution steps the message could not be successfully sent the 'TX Warn'
      | output is set to 1. Also, the message is expected to be sent every 50 ms approximatively. If this
      | condition is not met 5 times consecutively the 'TX Warn' output is set to 1.
  TX status : Inport
  TX delta time : Inport  Port=2
  Delta time limit : Constant  Value=2
  Delta time limit exceeded : RelationalOperator  RndMeth=Nearest  InputSameDT=on
  Mem{1..4} (4 alike) : Memory
  OR : Logic  Operator=OR
  Prev. msg. not sent : RelationalOperator  Operator=~=  RndMeth=Nearest  InputSameDT=on
  Prev. msg. sent value : Constant
  Rate Transition : RateTransition
  Rate Transition1 : RateTransition
  Warn : Logic  Inputs=5
  TX Warn : Outport
  wires:
  TX delta time/1 -> Rate Transition/1
  Delta time limit/1 -> Delta time limit exceeded/2
  Prev. msg. sent value/1 -> Prev. msg. not sent/2
  TX status/1 -> Rate Transition1/1
  Prev. msg. not sent/1 -> OR/1
  Delta time limit exceeded/1 -> OR/2
  OR/1 -> Mem1/1, Warn/1
  Mem1/1 -> Mem2/1, Warn/2
  Mem2/1 -> Mem3/1, Warn/3
  Mem3/1 -> Mem4/1, Warn/4
  Mem4/1 -> Warn/5
  Warn/1 -> TX Warn/1
  Rate Transition/1 -> Delta time limit exceeded/1
  Rate Transition1/1 -> Prev. msg. not sent/1

== system DR18E_Testpult/Ausgabe/Inverter TX/Umrichter Init/Transmit OK Detection1 ==
  note: This subsystem surveys if the sending of the TX message is successful and if it meets the
      | requirements concerning the regularity of the sending.
      |
      | If for 5 consecutive execution steps the message could not be successfully sent the 'TX Warn'
      | output is set to 1. Also, the message is expected to be sent every 50 ms approximatively. If this
      | condition is not met 5 times consecutively the 'TX Warn' output is set to 1.
  TX status : Inport
  TX delta time : Inport  Port=2
  Delta time limit : Constant  Value=2
  Delta time limit exceeded : RelationalOperator  RndMeth=Nearest  InputSameDT=on
  Mem{1..4} (4 alike) : Memory
  OR : Logic  Operator=OR
  Prev. msg. not sent : RelationalOperator  Operator=~=  RndMeth=Nearest  InputSameDT=on
  Prev. msg. sent value : Constant
  Rate Transition : RateTransition
  Rate Transition1 : RateTransition
  Warn : Logic  Inputs=5
  TX Warn : Outport
  wires:
  TX delta time/1 -> Rate Transition/1
  Delta time limit/1 -> Delta time limit exceeded/2
  Prev. msg. sent value/1 -> Prev. msg. not sent/2
  TX status/1 -> Rate Transition1/1
  Prev. msg. not sent/1 -> OR/1
  Delta time limit exceeded/1 -> OR/2
  OR/1 -> Mem1/1, Warn/1
  Mem1/1 -> Mem2/1, Warn/2
  Mem2/1 -> Mem3/1, Warn/3
  Mem3/1 -> Mem4/1, Warn/4
  Mem4/1 -> Warn/5
  Warn/1 -> TX Warn/1
  Rate Transition/1 -> Delta time limit exceeded/1
  Rate Transition1/1 -> Prev. msg. not sent/1

== system DR18E_Testpult/Eingabe Fahrzeug/BMS/RX Timeout Detection2/Subsystem ==
  TXStatus : Inport
  Timeout : Inport  Port=2
  Constant : Constant
  Constant1 : Constant  Value=0
  Constant2 : Constant
  Constant3 : Constant  Value=0
  Delay : Delay  DelayLength=1  InitialCondition=0
  Relational Operator : RelationalOperator  Operator=>  OutDataTypeStr=boolean  RndMeth=Nearest
  Sum : Sum  Inputs=|++
  Switch : Switch  Criteria=u2 > Threshold
  Switch1 : Switch  Criteria=u2 > Threshold
  Rampe : Outport
  RX Timeout Error : Outport  Port=2
  wires:
  TXStatus/1 -> Switch/2
  Delay/1 -> Sum/2
  Constant/1 -> Sum/1
  Sum/1 -> Switch/3
  Switch/1 -> Delay/1, Relational Operator/1, Rampe/1
  Constant1/1 -> Switch/1
  Constant2/1 -> Switch1/1
  Constant3/1 -> Switch1/3
  Switch1/1 -> RX Timeout Error/1
  Relational Operator/1 -> Switch1/2
  Timeout/1 -> Relational Operator/2

== system DR18E_Testpult/Eingabe Fahrzeug/BMS/STK1-5_Temp /RX Timeout Detection1 ==
  RX status : Inport
  Timeout (n Samples) : Inport  Port=2
  Subsystem : Subsystem  TreatAsAtomicUnit=on
  Terminator_4 : Terminator
  RX Timeout Error : Outport
  wires:
  RX status/1 -> Subsystem/1(TXStatus)
  Subsystem/1(Rampe) -> Terminator_4/1
  Subsystem/2(RX Timeout Error) -> RX Timeout Error/1  "RX Timeout"
  Timeout (n Samples)/1 -> Subsystem/2(Timeout)

== system DR18E_Testpult/Eingabe Fahrzeug/BMS/STK1-5_Temp /RX Timeout Detection10 ==
  RX status : Inport
  Timeout (n Samples) : Inport  Port=2
  Subsystem : Subsystem  TreatAsAtomicUnit=on
  Terminator_4 : Terminator
  RX Timeout Error : Outport
  wires:
  RX status/1 -> Subsystem/1(TXStatus)
  Subsystem/1(Rampe) -> Terminator_4/1
  Subsystem/2(RX Timeout Error) -> RX Timeout Error/1  "RX Timeout"
  Timeout (n Samples)/1 -> Subsystem/2(Timeout)

== system DR18E_Testpult/Eingabe Fahrzeug/BMS/STK1-5_Temp /RX Timeout Detection2 ==
  RX status : Inport
  Timeout (n Samples) : Inport  Port=2
  Subsystem : Subsystem  TreatAsAtomicUnit=on
  Terminator_4 : Terminator
  RX Timeout Error : Outport
  wires:
  RX status/1 -> Subsystem/1(TXStatus)
  Subsystem/1(Rampe) -> Terminator_4/1
  Subsystem/2(RX Timeout Error) -> RX Timeout Error/1  "RX Timeout"
  Timeout (n Samples)/1 -> Subsystem/2(Timeout)

== system DR18E_Testpult/Eingabe Fahrzeug/BMS/STK1-5_Temp /RX Timeout Detection3 ==
  RX status : Inport
  Timeout (n Samples) : Inport  Port=2
  Subsystem : Subsystem  TreatAsAtomicUnit=on
  Terminator_4 : Terminator
  RX Timeout Error : Outport
  wires:
  RX status/1 -> Subsystem/1(TXStatus)
  Subsystem/1(Rampe) -> Terminator_4/1
  Subsystem/2(RX Timeout Error) -> RX Timeout Error/1  "RX Timeout"
  Timeout (n Samples)/1 -> Subsystem/2(Timeout)

== system DR18E_Testpult/Eingabe Fahrzeug/BMS/STK1-5_Temp /RX Timeout Detection4 ==
  RX status : Inport
  Timeout (n Samples) : Inport  Port=2
  Subsystem : Subsystem  TreatAsAtomicUnit=on
  Terminator_4 : Terminator
  RX Timeout Error : Outport
  wires:
  RX status/1 -> Subsystem/1(TXStatus)
  Subsystem/1(Rampe) -> Terminator_4/1
  Subsystem/2(RX Timeout Error) -> RX Timeout Error/1  "RX Timeout"
  Timeout (n Samples)/1 -> Subsystem/2(Timeout)

== system DR18E_Testpult/Eingabe Fahrzeug/BMS/STK1-5_Temp /RX Timeout Detection5 ==
  RX status : Inport
  Timeout (n Samples) : Inport  Port=2
  Subsystem : Subsystem  TreatAsAtomicUnit=on
  Terminator_4 : Terminator
  RX Timeout Error : Outport
  wires:
  RX status/1 -> Subsystem/1(TXStatus)
  Subsystem/1(Rampe) -> Terminator_4/1
  Subsystem/2(RX Timeout Error) -> RX Timeout Error/1  "RX Timeout"
  Timeout (n Samples)/1 -> Subsystem/2(Timeout)

== system DR18E_Testpult/Eingabe Fahrzeug/BMS/STK1-5_Temp /RX Timeout Detection6 ==
  RX status : Inport
  Timeout (n Samples) : Inport  Port=2
  Subsystem : Subsystem  TreatAsAtomicUnit=on
  Terminator_4 : Terminator
  RX Timeout Error : Outport
  wires:
  RX status/1 -> Subsystem/1(TXStatus)
  Subsystem/1(Rampe) -> Terminator_4/1
  Subsystem/2(RX Timeout Error) -> RX Timeout Error/1  "RX Timeout"
  Timeout (n Samples)/1 -> Subsystem/2(Timeout)

== system DR18E_Testpult/Eingabe Fahrzeug/BMS/STK1-5_Temp /RX Timeout Detection7 ==
  RX status : Inport
  Timeout (n Samples) : Inport  Port=2
  Subsystem : Subsystem  TreatAsAtomicUnit=on
  Terminator_4 : Terminator
  RX Timeout Error : Outport
  wires:
  RX status/1 -> Subsystem/1(TXStatus)
  Subsystem/1(Rampe) -> Terminator_4/1
  Subsystem/2(RX Timeout Error) -> RX Timeout Error/1  "RX Timeout"
  Timeout (n Samples)/1 -> Subsystem/2(Timeout)
